simulink model "tank_level_sim"  (R2021b)
settings: Solver=VariableStepAuto  StartTime=0.0  StopTime=600  MaxStep=0.1  RelTol=1e-3  EnableMultiTasking=on
InitFcn:
  | warning off;
StopFcn:
  | warning on
  | 
  | addpath("~/ml-plot-utils")
  | 
  | figure(1); clf
  | 
  | % subplot(211)
  | % plot(r.time,r.data,y.time,y.data,'LineWidth',2)
  | % title('Response of closed-loop system')
  | % ylabel('r(t) , y(t)')
  | % xlabel('Time (s)')
  | % grid on
  | %
  | % subplot(212)
  | % plot(u.time,u.data,'LineWidth',2)
  | % title('Control action')
  | % ylabel('u(t)')
  | % xlabel('Time (s)')
  | % grid on
  | 
  | u_labels = ["$u(k)$" "$p(k)$"]
  | make_iorplot(y.data,y.time,[u.data p.data],r.data,u_labels)
undefined symbols (not defined in the file or in its folder): DiscIntNeverNeededParam
libraries: simulink x2
settings Model: Creator=Eric  LastModifiedBy=billtubbs
settings SolverCC: AlgebraicLoopSolver=TrustRegion
settings DataIOCC: LimitDataPoints=on  SaveFormat=Array  SignalLoggingSaveFormat=ModelDataLogs  SaveTime=off  ReturnWorkspaceOutputs=off
settings OptimizationCC: ExpressionDepthLimit=2147483647  LifeSpan=inf
settings DebuggingCC: UnderspecifiedInitializationDetection=Classic  MergeDetectMultiDrivingBlocksExec=none  SolverPrmCheckMsg=warning  FcnCallInpInsideContextMsg=warning  StateNameClashWarn=warning  SFUnexpectedBacktrackingDiag=warning  SFNoUnconditionalDefaultTransitionDiag=warning  SFExecutionAtInitializationDiag=none  SFMachineParentedDataDiag=warning  ArithmeticOperatorsInVariantConditions=warning
settings HardwareCC: ProdBitPerPointer=32  ProdBitPerSizeT=32  ProdBitPerPtrDiffT=32  ProdLargestAtomicFloat=None  ProdIntDivRoundTo=Undefined  ProdEndianess=Unspecified  ProdWordSize=32  ProdHWDeviceType=32-bit Generic
settings ModelReferenceCC: PropagateSignalLabelsOutOfModel=off
settings SFSimCC: SimUseLocalCustomCode=off  CustomCodeUndefinedFunction=UseInterfaceOnly
settings RTWCC: RTWUseLocalCustomCode=off
settings CodeAppCC: StateflowObjectComments=on
settings GRTTargetCC: TargetLangStandard=C89/C90 (ANSI)  CombineOutputUpdateFcns=off  GRTInterface=on
settings ConfigComp: CovMetricSettings=dw  CovSaveCumulativeToWorkspaceVar=on  CovSaveSingleToWorkspaceVar=on  CovExternalEMLEnable=off  CovSFcnEnable=off

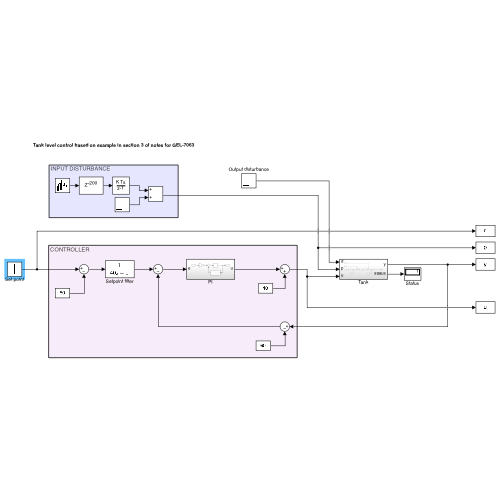
[thumbnail: Simulink's stored preview of the top-level diagram]
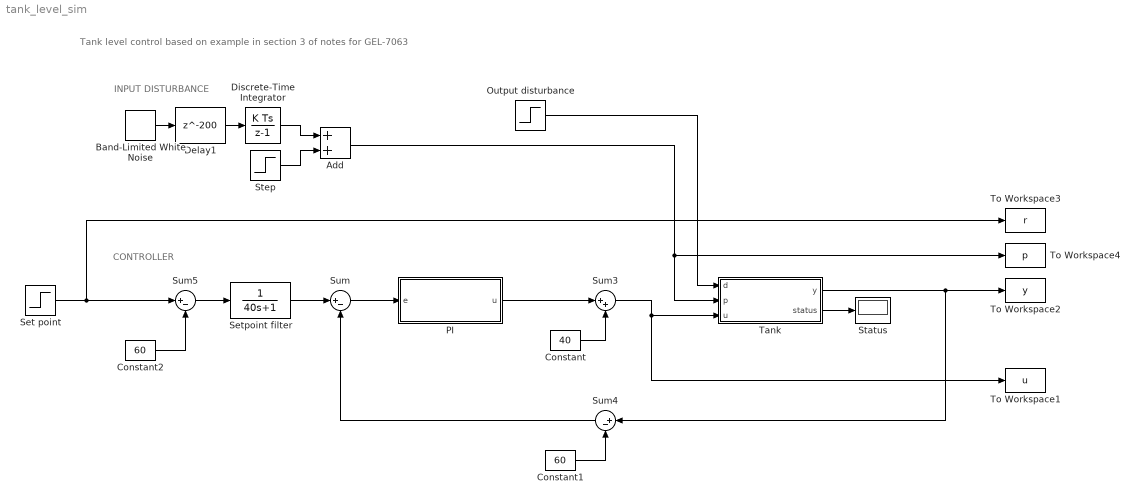
== system tank_level_sim ==
  note: INPUT DISTURBANCE
  note: Tank level control based on example in section 3 of notes for GEL-7063
  note: CONTROLLER
  Add : Sum
  Band-Limited White Noise : simulink/Sources/Band-Limited White Noise  Cov=[0.1]  Ts=1  seed=[23341]
  Constant : Constant  Value=40
  Constant1 : Constant  Value=60
  Constant2 : Constant  Value=60
  Delay1 : Delay  DelayLength=200  InputProcessing=Columns as channels (frame based)
  Discrete-Time Integrator : DiscreteIntegrator  gainval=1  SampleTime=-1  ICPrevOutput=DiscIntNeverNeededParam  ICPrevScaledInput=DiscIntNeverNeededParam
  Output disturbance : Step  After=0  SampleTime=0
  PI : Subsystem
  Set point : Step  Time=10  Before=60  After=70  SampleTime=0
  Setpoint filter : TransferFcn  Denominator=[40 1]
  Status : Display
  Step : Step  Time=300  After=0  SampleTime=0
  Sum : Sum  Inputs=|+-
  Sum3 : Sum  Inputs=|++
  Sum4 : Sum  Inputs=|+-
  Sum5 : Sum  Inputs=|+-
  Tank : Subsystem
  To Workspace1 : ToWorkspace  VariableName=u  SaveFormat=Timeseries  SampleTime=-1
  To Workspace2 : ToWorkspace  VariableName=y  SaveFormat=Timeseries  SampleTime=-1
  To Workspace3 : ToWorkspace  VariableName=r  SaveFormat=Timeseries  SampleTime=-1
  To Workspace4 : ToWorkspace  VariableName=p  SaveFormat=Timeseries  SampleTime=-1
  wires:
  Sum3/1 -> To Workspace1/1, Tank/3(u)
  Set point/1 -> To Workspace3/1, Sum5/1
  Add/1 -> Tank/2(p), To Workspace4/1
  Sum/1 -> PI/1(e)
  Setpoint filter/1 -> Sum/1
  PI/1(u) -> Sum3/1
  Constant/1 -> Sum3/2
  Constant1/1 -> Sum4/2
  Tank/1(y) -> To Workspace2/1, Sum4/1
  Band-Limited White Noise/1 -> Delay1/1
  Discrete-Time Integrator/1 -> Add/1
  Step/1 -> Add/2
  Delay1/1 -> Discrete-Time Integrator/1
  Tank/2(status) -> Status/1
  Sum4/1 -> Sum/2
  Constant2/1 -> Sum5/2
  Sum5/1 -> Setpoint filter/1
  Output disturbance/1 -> Tank/1(d)

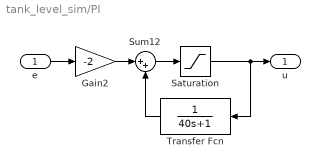
== system tank_level_sim/PI ==
  e : Inport
  Gain2 : Gain  Gain=-2
  Saturation : Saturate  UpperLimit=60  LowerLimit=-40
  Sum12 : Sum  Inputs=|++
  Transfer Fcn : TransferFcn  Numerator=1  Denominator=[40 1]
  u : Outport
  wires:
  e/1 -> Gain2/1
  Transfer Fcn/1 -> Sum12/2
  Gain2/1 -> Sum12/1
  Sum12/1 -> Saturation/1
  Saturation/1 -> Transfer Fcn/1, u/1

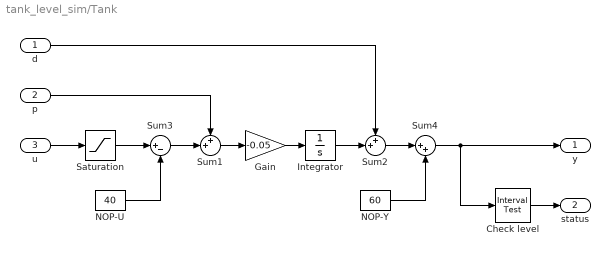
== system tank_level_sim/Tank ==
  d : Inport
  p : Inport  Port=2
  u : Inport  Port=3
  Check level : simulink/Logic and Bit Operations/Interval Test  IntervalClosedRight=on  uplimit=100  IntervalClosedLeft=on  lowlimit=0  OutDataTypeStr=boolean
  Gain : Gain  Gain=-0.05
  Integrator : Integrator
  NOP-U : Constant  Value=40
  NOP-Y : Constant  Value=60
  Saturation : Saturate  UpperLimit=100  LowerLimit=0
  Sum1 : Sum  Inputs=++|
  Sum2 : Sum  Inputs=++|
  Sum3 : Sum  Inputs=|+-
  Sum4 : Sum  Inputs=|++
  y : Outport
  status : Outport  Port=2
  wires:
  d/1 -> Sum2/1
  Gain/1 -> Integrator/1
  p/1 -> Sum1/1
  Integrator/1 -> Sum2/2
  Sum2/1 -> Sum4/1
  u/1 -> Saturation/1
  Sum1/1 -> Gain/1
  NOP-U/1 -> Sum3/2
  Saturation/1 -> Sum3/1
  Sum3/1 -> Sum1/2
  NOP-Y/1 -> Sum4/2
  Sum4/1 -> y/1, Check level/1
  Check level/1 -> status/1
